simulink model "untitled1"  (R2018b)
settings: Solver=FixedStepAuto  StartTime=0.0  StopTime=10  RelTol=1e-3  EnableMultiTasking=on
libraries: embdlinuxlib x11
settings Model: Creator=DELL  LastModifiedBy=DELL
settings SolverCC: PositivePriorityOrder=on
settings OptimizationCC: EnhancedBackFolding=on  PassReuseOutputArgsAs=Individual arguments  MaxStackSize=64  OptimizeBlockOrder=speed  DifferentSizesBufferReuse=on  OptimizationCustomize=off
settings DebuggingCC: ParameterTunabilityLossMsg=error
settings HardwareCC: ProdBitPerPointer=32  ProdBitPerSizeT=32  ProdBitPerPtrDiffT=32  ProdLargestAtomicInteger=Long  ProdLargestAtomicFloat=Double  ProdWordSize=32  ProdHWDeviceType=ARM Compatible->ARM Cortex
settings SFSimCC: MATLABDynamicMemAlloc=off
settings RTWCC: SystemTargetFile=ert.tlc  HardwareBoard=Raspberry Pi  TLCOptions="-aInlineSetEventsForThisBaseRateFcn=TLC_FALSE -aSuppressMultiTaskScheduler=TLC_FALSE  -aRateBasedStepFcn=0"  TemplateMakefile=ert_default_tmf  GenerateReport=on  Toolchain=GNU GCC Raspberry Pi  BuildConfiguration=Faster Runs  IncludeHyperlinkInReport=on  LaunchReport=on  GenerateTraceInfo=on  GenerateTraceReport=on  GenerateTraceReportSl=on  GenerateTraceReportSf=on  GenerateTraceReportEml=on
settings CodeAppCC: ForceParamTrailComments=on  IgnoreCustomStorageClasses=off  OperatorAnnotations=on  SimulinkDataObjDesc=on  SFDataObjDesc=on  InsertBlockDesc=on
settings ERTTargetCC: SupportVariableSizeSignals=on

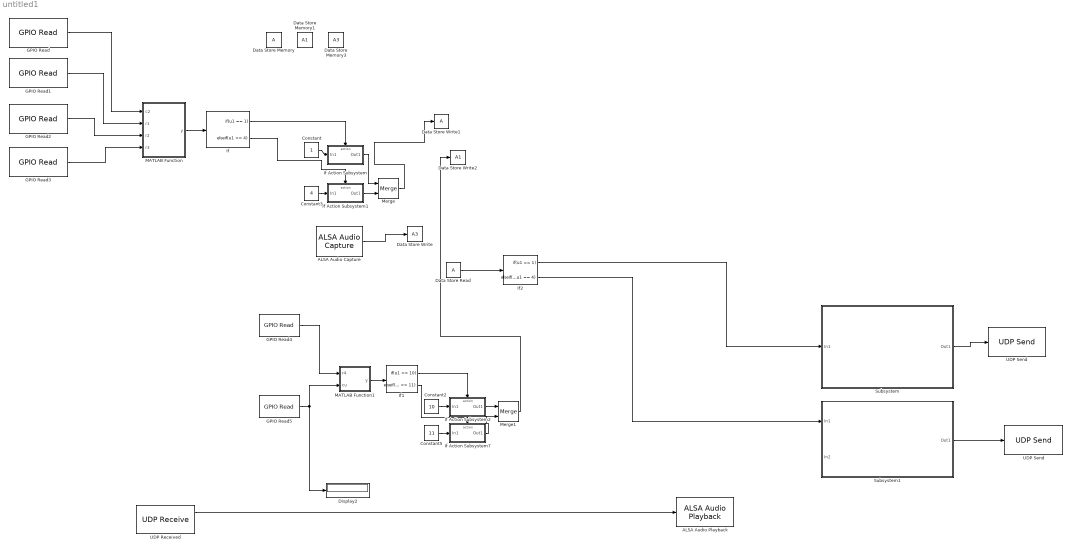
== system untitled1 ==
  ALSA Audio Capture : embdlinuxlib/ALSA Audio Capture  deviceStr='hw:1,0'  DataBitDepth=16-bit integer  numberOfChannels=1  sampleRateEnum=44100  frameSize=4410  QueueDuration=0.5  blockPlatform=Raspberry Pi
      settings: SourceProductName=Simulink Support Package for Raspberry Pi Hardware  SourceProductBaseCode=RASPPI
  ALSA Audio Playback : embdlinuxlib/ALSA Audio Playback  deviceStr='hw:0,0'  sampleRateEnum=44100  queueDuration=0.5  blockPlatform=Raspberry Pi
      settings: SourceProductName=Simulink Support Package for Raspberry Pi Hardware  SourceProductBaseCode=RASPPI
  Constant : Constant
  Constant2 : Constant  Value=10
  Constant3 : Constant  Value=4
  Constant5 : Constant  Value=11
  Data Store Memory : DataStoreMemory  ReadBeforeWriteMsg=warning  WriteAfterWriteMsg=warning  WriteAfterReadMsg=warning  ShowAdditionalParam=off
  Data Store Memory1 : DataStoreMemory  DataStoreName=A1  ReadBeforeWriteMsg=warning  WriteAfterWriteMsg=warning  WriteAfterReadMsg=warning  ShowAdditionalParam=off
  Data Store Memory3 : DataStoreMemory  DataStoreName=A3  ReadBeforeWriteMsg=warning  WriteAfterWriteMsg=warning  WriteAfterReadMsg=warning  ShowAdditionalParam=off  Dimensions=[4410,1]
  Data Store Read : DataStoreRead
  Data Store Write : DataStoreWrite  DataStoreName=A3
  Data Store Write1 : DataStoreWrite
  Data Store Write2 : DataStoreWrite  DataStoreName=A1
  Display2 : Display
  GPIO Read : embdlinuxlib/GPIO Read  board=Pi 3 Model B+  gpio=22  internalResistor=Off  sampleTime=0.1  direction=Input  blockPlatform=Raspberry Pi
      settings: SourceProductName=Simulink Support Package for Raspberry Pi Hardware  SourceProductBaseCode=RASPPI
  GPIO Read1 : embdlinuxlib/GPIO Read  board=Pi 3 Model B+  gpio=27  internalResistor=Off  sampleTime=0.1  direction=Input  blockPlatform=Raspberry Pi
      settings: SourceProductName=Simulink Support Package for Raspberry Pi Hardware  SourceProductBaseCode=RASPPI
  GPIO Read2 : embdlinuxlib/GPIO Read  board=Pi 3 Model B+  gpio=23  internalResistor=Off  sampleTime=0.1  direction=Input  blockPlatform=Raspberry Pi
      settings: SourceProductName=Simulink Support Package for Raspberry Pi Hardware  SourceProductBaseCode=RASPPI
  GPIO Read3 : embdlinuxlib/GPIO Read  board=Pi 3 Model B+  gpio=24  internalResistor=Off  sampleTime=0.1  direction=Input  blockPlatform=Raspberry Pi
      settings: SourceProductName=Simulink Support Package for Raspberry Pi Hardware  SourceProductBaseCode=RASPPI
  GPIO Read4 : embdlinuxlib/GPIO Read  board=Pi 3 Model B+  gpio=25  internalResistor=Off  sampleTime=0.1  direction=Input  blockPlatform=Raspberry Pi
      settings: SourceProductName=Simulink Support Package for Raspberry Pi Hardware  SourceProductBaseCode=RASPPI
  GPIO Read5 : embdlinuxlib/GPIO Read  board=Pi 3 Model B+  gpio=17  internalResistor=Off  sampleTime=0.1  direction=Input  blockPlatform=Raspberry Pi
      settings: SourceProductName=Simulink Support Package for Raspberry Pi Hardware  SourceProductBaseCode=RASPPI
  If : If  IfExpression=u1 == 1  ElseIfExpressions=u1 == 4  ShowElse=off
  If Action Subsystem : Subsystem  TreatAsAtomicUnit=on
  If Action Subsystem1 : Subsystem  TreatAsAtomicUnit=on
  If Action Subsystem2 : Subsystem  TreatAsAtomicUnit=on
  If Action Subsystem7 : Subsystem  TreatAsAtomicUnit=on
  If1 : If  IfExpression=u1 == 10  ElseIfExpressions=u1 == 11  ShowElse=off
  If2 : If  IfExpression=u1 == 1  ElseIfExpressions=u1 == 4  ShowElse=off
  MATLAB Function : MATLAB Function  TreatAsAtomicUnit=on
  MATLAB Function1 : MATLAB Function  TreatAsAtomicUnit=on
  Merge : Merge
  Merge1 : Merge
  Subsystem : Subsystem
  Subsystem1 : Subsystem
  UDP Received : embdlinuxlib/UDP Receive  localURL='0.0.0.0'  localPort=25000  remoteURL='0.0.0.0'  remotePort=-1  recvBufferSize=8192  signalDatatype=int16  dims=4410  isVarSize=off  showBlockingTime=off  blockingTime=0  sampletime=0.1  blockPlatform=Raspberry Pi
      settings: SourceProductName=Simulink Support Package for Raspberry Pi Hardware  SourceProductBaseCode=RASPPI
  UDP Send : embdlinuxlib/UDP Send  remoteURL='192.168.24.118'  remotePort=25000  localURL='255.255.255.255'  localPortSource=Automatically determine  localPort=-1  sampletime=-1  blockPlatform=Raspberry Pi  separateLengthPort=0
      settings: SourceProductName=Simulink Support Package for Raspberry Pi Hardware  SourceProductBaseCode=RASPPI
  "UDP Send " : embdlinuxlib/UDP Send  remoteURL='192.168.24.133'  remotePort=25000  localURL='255.255.255.255'  localPortSource=Automatically determine  localPort=-1  sampletime=-1  blockPlatform=Raspberry Pi  separateLengthPort=0
      settings: SourceProductName=Simulink Support Package for Raspberry Pi Hardware  SourceProductBaseCode=RASPPI
  wires:
  GPIO Read/1 -> MATLAB Function/1(c2)
  GPIO Read1/1 -> MATLAB Function/2(r1)
  Data Store Read/1 -> If2/1
  If/1 -> If Action Subsystem/Action
  Constant/1 -> If Action Subsystem/1(In1)
  If Action Subsystem/1(Out1) -> Merge/1
  If Action Subsystem1/1(Out1) -> Merge/2
  Merge/1 -> Data Store Write1/1
  If/2 -> If Action Subsystem1/Action
  GPIO Read2/1 -> MATLAB Function/3(r2)
  MATLAB Function/1(y) -> If/1
  GPIO Read4/1 -> MATLAB Function1/1(r4)
  MATLAB Function1/1(y) -> If1/1
  If1/1 -> If Action Subsystem2/Action
  Constant2/1 -> If Action Subsystem2/1(In1)
  GPIO Read3/1 -> MATLAB Function/4(r3)
  GPIO Read5/1 -> Display2/1, MATLAB Function1/2(cu)
  Constant5/1 -> If Action Subsystem7/1(In1)
  If1/2 -> If Action Subsystem7/Action
  If Action Subsystem2/1(Out1) -> Merge1/1
  If Action Subsystem7/1(Out1) -> Merge1/2
  Merge1/1 -> Data Store Write2/1
  Constant3/1 -> If Action Subsystem1/1(In1)
  ALSA Audio Capture/1 -> Data Store Write/1
  If2/1 -> Subsystem/1(In1)
  Subsystem/1(Out1) -> "UDP Send "/1
  If2/2 -> Subsystem1/1(In1)
  Subsystem1/1(Out1) -> UDP Send/1
  UDP Received/1 -> ALSA Audio Playback/1

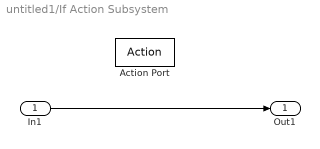
== system untitled1/If Action Subsystem ==
  In1 : Inport
  Action Port : ActionPort  InitializeStates=reset  ActionType=then
  Out1 : Outport
  wires:
  In1/1 -> Out1/1

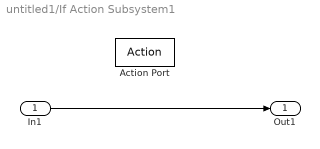
== system untitled1/If Action Subsystem1 ==
  In1 : Inport
  Action Port : ActionPort  InitializeStates=reset  ActionType=elseif
  Out1 : Outport
  wires:
  In1/1 -> Out1/1

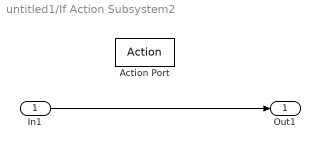
== system untitled1/If Action Subsystem2 ==
  In1 : Inport
  Action Port : ActionPort  InitializeStates=reset  ActionType=then
  Out1 : Outport
  wires:
  In1/1 -> Out1/1

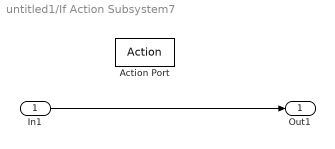
== system untitled1/If Action Subsystem7 ==
  In1 : Inport
  Action Port : ActionPort  InitializeStates=reset  ActionType=elseif
  Out1 : Outport
  wires:
  In1/1 -> Out1/1

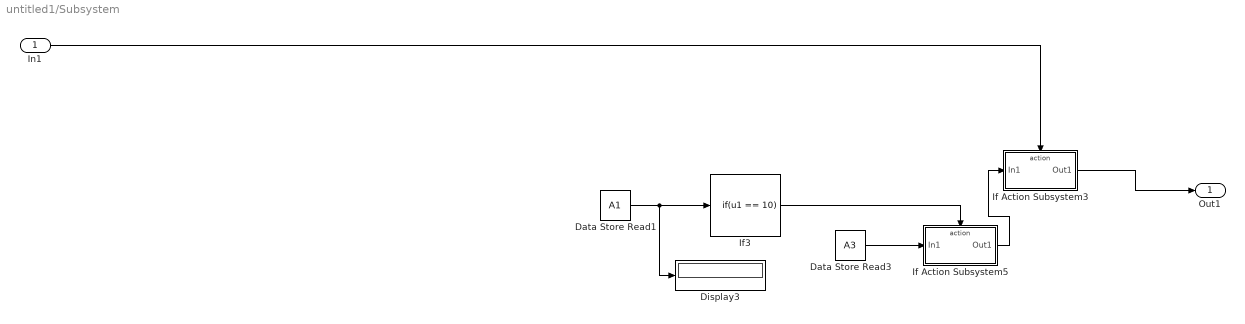
== system untitled1/Subsystem ==
  In1 : Inport
  Data Store Read1 : DataStoreRead  DataStoreName=A1
  Data Store Read3 : DataStoreRead  DataStoreName=A3
  Display3 : Display
  If Action Subsystem3 : Subsystem  TreatAsAtomicUnit=on
  If Action Subsystem5 : Subsystem  TreatAsAtomicUnit=on
  If3 : If  IfExpression=u1 == 10  ShowElse=off
  Out1 : Outport
  wires:
  Data Store Read3/1 -> If Action Subsystem5/1(In1)
  Data Store Read1/1 -> Display3/1, If3/1
  If Action Subsystem5/1(Out1) -> If Action Subsystem3/1(In1)
  In1/1 -> If Action Subsystem3/Action
  If3/1 -> If Action Subsystem5/Action
  If Action Subsystem3/1(Out1) -> Out1/1

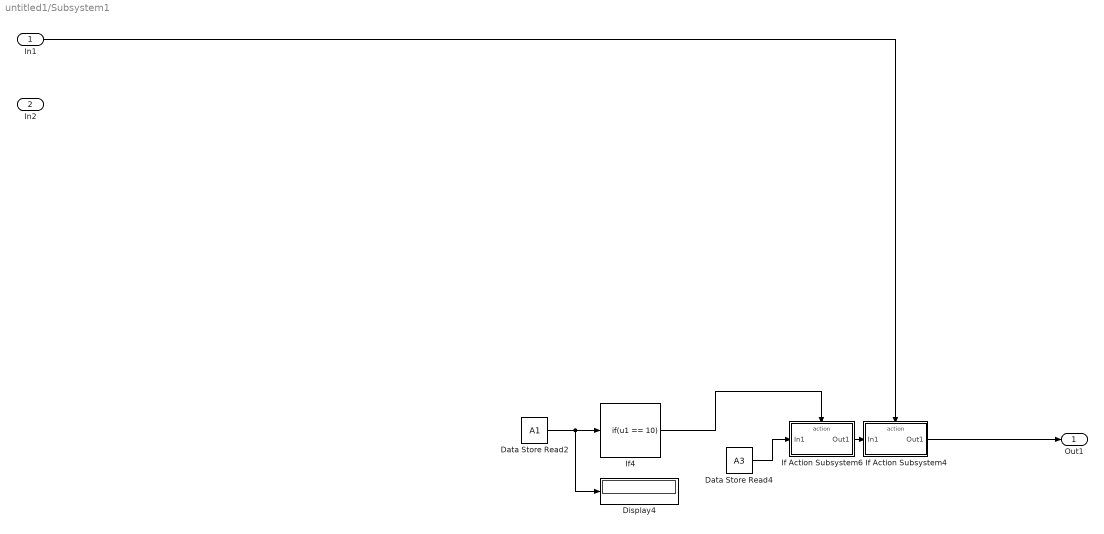
== system untitled1/Subsystem1 ==
  In1 : Inport
  In2 : Inport  Port=2
  Data Store Read2 : DataStoreRead  DataStoreName=A1
  Data Store Read4 : DataStoreRead  DataStoreName=A3
  Display4 : Display
  If Action Subsystem4 : Subsystem  TreatAsAtomicUnit=on
  If Action Subsystem6 : Subsystem  TreatAsAtomicUnit=on
  If4 : If  IfExpression=u1 == 10  ShowElse=off
  Out1 : Outport
  wires:
  In1/1 -> If Action Subsystem4/Action
  Data Store Read2/1 -> Display4/1, If4/1
  Data Store Read4/1 -> If Action Subsystem6/1(In1)
  If4/1 -> If Action Subsystem6/Action
  If Action Subsystem6/1(Out1) -> If Action Subsystem4/1(In1)
  If Action Subsystem4/1(Out1) -> Out1/1

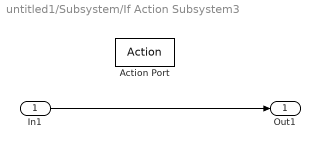
== system untitled1/Subsystem/If Action Subsystem3 ==
  In1 : Inport
  Action Port : ActionPort  InitializeStates=reset  ActionType=then
  Out1 : Outport
  wires:
  In1/1 -> Out1/1

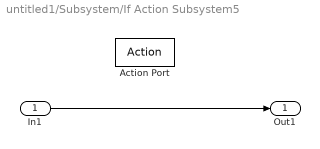
== system untitled1/Subsystem/If Action Subsystem5 ==
  In1 : Inport
  Action Port : ActionPort  InitializeStates=reset  ActionType=then
  Out1 : Outport
  wires:
  In1/1 -> Out1/1

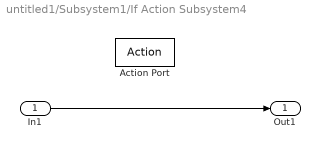
== system untitled1/Subsystem1/If Action Subsystem4 ==
  In1 : Inport
  Action Port : ActionPort  InitializeStates=reset  ActionType=elseif
  Out1 : Outport
  wires:
  In1/1 -> Out1/1

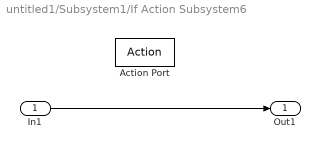
== system untitled1/Subsystem1/If Action Subsystem6 ==
  In1 : Inport
  Action Port : ActionPort  InitializeStates=reset  ActionType=then
  Out1 : Outport
  wires:
  In1/1 -> Out1/1

== matlab function untitled1/MATLAB Function1 ==
  data: r4 input; y output; cu input
function y = fcn(r4,cu)
if(r4==logical(1))
    y=10;
elseif(cu==logical(1))
    y=11;
else
   y=50;
end

== matlab function untitled1/MATLAB Function ==
  data: c2 input; r1 input; y output; r2 input; r3 input
function y = fcn(c2,r1,r2,r3)
if(c2==logical(1) && r2==logical(1))
    y=1;
elseif(c2==logical(1) && r1==logical(1))
    y=4;
elseif(c2==logical(1) && r3==logical(1))
    y=7;  
else
   y=50;
end
